simulink model "QRF_fp"  (R2019a)
settings: Solver=VariableStepAuto  StartTime=0.0  StopTime=simulation_stop_time  RelTol=1e-3
values from neighbouring files (symbols this model uses):
  sample_time = 1 / input_sample_freq    (= 1e-06)    [project_main.m]
libraries: simulink x5
settings Model: SimulationMode=accelerator  Creator=ASUAD\sasiddi8  LastModifiedBy=ASUAD\sasiddi8
settings OptimizationCC: BlockReduction=off  ConditionallyExecuteInputs=off  DefaultParameterBehavior=Inlined
settings DebuggingCC: SignalRangeChecking=error  AlgebraicLoopMsg=error  IntegerOverflowMsg=none  ParameterDowncastMsg=none  ParameterOverflowMsg=none  ParameterPrecisionLossMsg=none  IntegerSaturationMsg=none
settings HardwareCC: ProdBitPerPointer=32  ProdBitPerSizeT=32  ProdBitPerPtrDiffT=32  ProdLargestAtomicFloat=None  ProdIntDivRoundTo=Undefined  ProdEndianess=Unspecified  ProdWordSize=32  ProdHWDeviceType=ASIC/FPGA->ASIC/FPGA  TargetBitPerLong=64  TargetBitPerPointer=64  TargetBitPerSizeT=64  TargetBitPerPtrDiffT=64  TargetLongLongMode=on  TargetIntDivRoundTo=Zero  TargetEndianess=LittleEndian  TargetWordSize=64  TargetHWDeviceType=Custom Processor->MATLAB Host Computer  ProdEqTarget=off

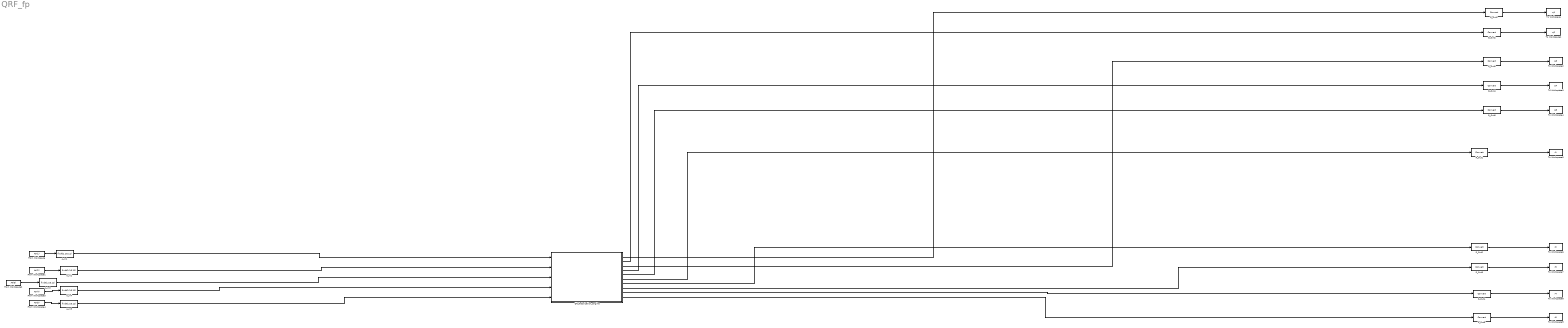
== system QRF_fp ==
  A_In{1..5} (5 alike) : DataTypeConversion  OutDataTypeStr=fixdt(1,16,11)
  From Workspace : FromWorkspace  VariableName=AtI(1)  OutDataTypeStr=double  SampleTime=sample_time  Interpolate=off  OutputAfterFinalValue=Holding final value
  From Workspace1 : FromWorkspace  VariableName=AtI(2)  OutDataTypeStr=double  SampleTime=sample_time  Interpolate=off  OutputAfterFinalValue=Holding final value
  From Workspace2 : FromWorkspace  VariableName=AtI(3)  OutDataTypeStr=double  SampleTime=sample_time  Interpolate=off  OutputAfterFinalValue=Holding final value
  From Workspace3 : FromWorkspace  VariableName=AtI(4)  OutDataTypeStr=double  SampleTime=sample_time  Interpolate=off  OutputAfterFinalValue=Holding final value
  From Workspace4 : FromWorkspace  VariableName=AtI(5)  OutDataTypeStr=double  SampleTime=sample_time  Interpolate=off  OutputAfterFinalValue=Holding final value
  QR_factorization_engine : Subsystem
  Q_Out{1..5} (5 alike) : DataTypeConversion
  R_Out{1..5} (5 alike) : DataTypeConversion
  To Workspace : ToWorkspace  VariableName=q1  SaveFormat=Structure With Time  SampleTime=-1
  To Workspace1 : ToWorkspace  VariableName=q2  SaveFormat=Structure With Time  SampleTime=-1
  To Workspace2 : ToWorkspace  VariableName=q3  SaveFormat=Structure With Time  SampleTime=-1
  To Workspace3 : ToWorkspace  VariableName=q4  SaveFormat=Structure With Time  SampleTime=-1
  To Workspace4 : ToWorkspace  VariableName=q5  SaveFormat=Structure With Time  SampleTime=-1
  To Workspace5 : ToWorkspace  VariableName=r1  SaveFormat=Structure With Time  SampleTime=-1
  To Workspace6 : ToWorkspace  VariableName=r2  SaveFormat=Structure With Time  SampleTime=-1
  To Workspace7 : ToWorkspace  VariableName=r3  SaveFormat=Structure With Time  SampleTime=-1
  To Workspace8 : ToWorkspace  VariableName=r4  SaveFormat=Structure With Time  SampleTime=-1
  To Workspace9 : ToWorkspace  VariableName=r5  SaveFormat=Structure With Time  SampleTime=-1
  wires:
  Q_Out1/1 -> To Workspace/1
  Q_Out2/1 -> To Workspace1/1
  Q_Out3/1 -> To Workspace2/1
  Q_Out4/1 -> To Workspace3/1
  Q_Out5/1 -> To Workspace4/1
  R_Out1/1 -> To Workspace5/1
  R_Out2/1 -> To Workspace6/1
  R_Out3/1 -> To Workspace7/1
  R_Out4/1 -> To Workspace8/1
  R_Out5/1 -> To Workspace9/1
  From Workspace/1 -> A_In1/1
  From Workspace1/1 -> A_In2/1
  From Workspace2/1 -> A_In3/1
  From Workspace3/1 -> A_In4/1
  From Workspace4/1 -> A_In5/1
  A_In1/1 -> QR_factorization_engine/1(In1)
  A_In2/1 -> QR_factorization_engine/2(In2)
  A_In3/1 -> QR_factorization_engine/3(In3)
  A_In4/1 -> QR_factorization_engine/4(In4)
  A_In5/1 -> QR_factorization_engine/5(In5)
  QR_factorization_engine/1(Out1) -> Q_Out1/1
  QR_factorization_engine/2(Out2) -> Q_Out2/1
  QR_factorization_engine/3(Out3) -> Q_Out3/1
  QR_factorization_engine/4(Out4) -> Q_Out4/1
  QR_factorization_engine/5(Out5) -> Q_Out5/1
  QR_factorization_engine/6(Out6) -> R_Out1/1
  QR_factorization_engine/7(Out7) -> R_Out2/1
  QR_factorization_engine/8(Out8) -> R_Out3/1
  QR_factorization_engine/9(Out9) -> R_Out4/1
  QR_factorization_engine/10(Out10) -> R_Out5/1

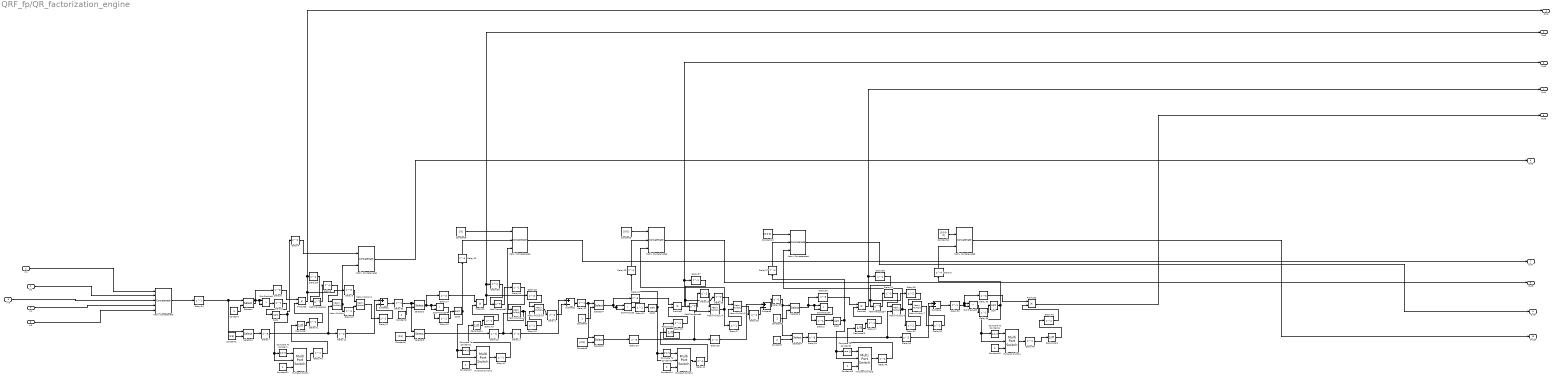
== system QRF_fp/QR_factorization_engine ==
  In1 : Inport
  In2 : Inport  Port=2
  In3 : Inport  Port=3
  In4 : Inport  Port=4
  In5 : Inport  Port=5
  Compare To Constant{,1..4} (5 alike) : simulink/Logic and Bit Operations/Compare To Constant  relop===  const=0  OutDataTypeStr=boolean
  Constant{,2,4,6} (4 alike) : Constant  VectorParams1D=off  OutDataTypeStr=fixdt(0,8,0)  SampleTime=sample_time
  Constant1 : Constant  Value=[2:5]  VectorParams1D=off  OutDataTypeStr=fixdt(0,8,0)  SampleTime=sample_time
  Constant10 : Constant  Value=[0 0 0]  VectorParams1D=off  OutDataTypeStr=fixdt(1,32,26)  SampleTime=sample_time
  Constant11 : Constant  Value=[0 0 0 0]  VectorParams1D=off  OutDataTypeStr=fixdt(0,16,12)  SampleTime=sample_time
  Constant{12..16} (5 alike) : Constant  VectorParams1D=off  OutDataTypeStr=fixdt(0,16,15)  SampleTime=sample_time
  Constant3 : Constant  Value=[2:4]  VectorParams1D=off  OutDataTypeStr=fixdt(0,8,0)  SampleTime=sample_time
  Constant5 : Constant  Value=[2:3]  VectorParams1D=off  OutDataTypeStr=fixdt(0,8,0)  SampleTime=sample_time
  Constant7 : Constant  Value=2  VectorParams1D=off  OutDataTypeStr=fixdt(0,8,0)  SampleTime=sample_time
  Constant8 : Constant  Value=[0]  VectorParams1D=off  OutDataTypeStr=fixdt(1,32,26)  SampleTime=sample_time
  Constant9 : Constant  Value=[0 0]  VectorParams1D=off  OutDataTypeStr=fixdt(1,32,26)  SampleTime=sample_time
  Delay{1..2,5,8,10,12..13,15,19,21,23,27..28,31..33,38,40..58} (36 alike) : Delay  DelayLength=1  InitialCondition=0
  Delay{11,17,25..26,35..36} (6 alike) : Delay  InitialCondition=0
  Delay{6,9,14,18,22,30,39} (7 alike) : Delay  DelayLength=3  InitialCondition=0
  Delay{7,16,24,34} (4 alike) : Delay  DelayLength=5  InitialCondition=0
  Delay{3..4,20,29,37} (5 alike) : Delay  DelayLength=4  InitialCondition=0
  Dot Product{1..4} (4 alike) : DotProduct  OutDataTypeStr=fixdt(0,32,23)
  Dot Product5 : DotProduct  OutDataTypeStr=fixdt(0,32,24)
  MathTranspose{1..4} (4 alike) : Math  Operator=transpose  OutDataTypeStr=double  SaturateOnIntegerOverflow=on
  Matrix Concatenate : Concatenate  NumInputs=5  Mode=Multidimensional array  ConcatenateDimension=2
  Matrix Concatenate1 : Concatenate  Mode=Multidimensional array  ConcatenateDimension=2
  Matrix Concatenate2 : Concatenate  NumInputs=3  Mode=Multidimensional array  ConcatenateDimension=2
  Matrix Concatenate3 : Concatenate  NumInputs=3  Mode=Multidimensional array  ConcatenateDimension=2
  Matrix Concatenate4 : Concatenate  NumInputs=3  Mode=Multidimensional array  ConcatenateDimension=2
  Matrix Concatenate5 : Concatenate  Mode=Multidimensional array  ConcatenateDimension=2
  MatrixMultiply{,2,4,6} (4 alike) : Product  Multiplication=Matrix(*)  OutDataTypeStr=fixdt(1,32,26)
  MatrixMultiply1 : Product  Multiplication=Matrix(*)  OutDataTypeStr=fixdt(1,16,11)
  MatrixMultiply3 : Product  Multiplication=Matrix(*)  OutDataTypeStr=fixdt(1,16,11)
  MatrixMultiply5 : Product  Multiplication=Matrix(*)  OutDataTypeStr=fixdt(1,16,11)
  MatrixMultiply7 : Product  Multiplication=Matrix(*)  OutDataTypeStr=fixdt(1,32,27)
  Multiport Switch{,1..3} (4 alike) : MultiPortSwitch  DataPortOrder=Zero-based contiguous  Inputs=2  zeroidx=on  OutDataTypeStr=fixdt(0,16,11)
  Multiport Switch4 : MultiPortSwitch  DataPortOrder=Zero-based contiguous  Inputs=2  zeroidx=on  OutDataTypeStr=fixdt(0,16,12)
  Product{1..5} (5 alike) : Product  OutDataTypeStr=fixdt(1,16,15)
  Reciprocal : Product  Inputs=/  OutDataTypeStr=fixdt(0,32,31)  SaturateOnIntegerOverflow=on  RndMeth=Zero
  Reciprocal1 : Product  Inputs=/  OutDataTypeStr=fixdt(0,32,31)  SaturateOnIntegerOverflow=on  RndMeth=Zero
  Reciprocal2 : Product  Inputs=/  OutDataTypeStr=fixdt(0,32,30)  SaturateOnIntegerOverflow=on  RndMeth=Zero
  Reciprocal3 : Product  Inputs=/  OutDataTypeStr=fixdt(0,32,29)  SaturateOnIntegerOverflow=on  RndMeth=Zero
  Reciprocal4 : Product  Inputs=/  OutDataTypeStr=fixdt(0,32,25)  SaturateOnIntegerOverflow=on  RndMeth=Zero
  Selector{,1..7} (8 alike) : Selector  NumberOfDimensions=2  InputPortWidth=3  IndexOptions=Select all,Index vector (port)  Indices=[1 3],1  OutputSizes=1,1
  Sqrt : Sqrt  OutDataTypeStr=fixdt(0,16,12)  SaturateOnIntegerOverflow=on
  Sqrt{1..4} (4 alike) : Sqrt  OutDataTypeStr=fixdt(1,32,26)  SaturateOnIntegerOverflow=on
  Subtract1 : Sum  Inputs=+-  AccumDataTypeStr=fixdt(1,32,27)  OutDataTypeStr=fixdt(1,16,11)
  Subtract2 : Sum  Inputs=+-  AccumDataTypeStr=fixdt(1,32,27)  OutDataTypeStr=fixdt(1,16,11)
  Subtract3 : Sum  Inputs=+-  AccumDataTypeStr=fixdt(1,32,27)  OutDataTypeStr=fixdt(1,16,11)
  Subtract4 : Sum  Inputs=+-  AccumDataTypeStr=fixdt(1,32,27)  OutDataTypeStr=fixdt(1,32,27)
  Out1 : Outport
  Out2 : Outport  Port=2
  Out3 : Outport  Port=3
  Out4 : Outport  Port=4
  Out5 : Outport  Port=5
  Out6 : Outport  Port=6
  Out7 : Outport  Port=7
  Out8 : Outport  Port=8
  Out9 : Outport  Port=9
  Out10 : Outport  Port=10
  wires:
  Matrix Concatenate2/1 -> Out7/1
  Compare To Constant/1 -> Multiport Switch/1
  Constant4/1 -> Selector4/2
  Matrix Concatenate3/1 -> Out8/1
  In3/1 -> Matrix Concatenate/3
  MathTranspose2/1 -> Delay15/1
  Compare To Constant2/1 -> Multiport Switch2/1
  Constant8/1 -> Matrix Concatenate2/1
  Selector6/1 -> Dot Product4/2, Dot Product4/1, Delay30/1
  Constant6/1 -> Selector6/2
  Constant16/1 -> Multiport Switch4/3
  MathTranspose3/1 -> Delay23/1
  Matrix Concatenate/1 -> Delay54/1
  Selector7/1 -> Delay34/1
  Constant11/1 -> Matrix Concatenate5/1
  Compare To Constant4/1 -> Multiport Switch4/1
  Selector2/1 -> Dot Product2/2, Dot Product2/1, Delay14/1
  Sqrt1/1 -> Multiport Switch3/2, Compare To Constant3/1, Delay37/1
  Compare To Constant1/1 -> Multiport Switch1/1
  Constant2/1 -> Selector2/2
  In4/1 -> Matrix Concatenate/4
  Sqrt4/1 -> Multiport Switch/2, Compare To Constant/1, Delay4/1
  Sqrt3/1 -> Multiport Switch1/2, Compare To Constant1/1, Delay20/1
  Product4/1 -> Out4/1, Delay58/1
  Product2/1 -> Delay57/1, Out3/1
  MatrixMultiply6/1 -> Delay32/1, Matrix Concatenate4/3
  Constant3/1 -> Selector3/2
  Constant10/1 -> Matrix Concatenate4/1
  Constant12/1 -> Multiport Switch/3
  In1/1 -> Matrix Concatenate/1
  Sqrt/1 -> Multiport Switch4/2, Compare To Constant4/1, Delay3/1
  MatrixMultiply5/1 -> Delay28/1
  Constant1/1 -> Selector1/2
  Selector4/1 -> Dot Product3/1, Dot Product3/2, Delay22/1
  Matrix Concatenate1/1 -> Out6/1
  Selector/1 -> Delay6/1, Dot Product1/2, Dot Product1/1
  In5/1 -> Matrix Concatenate/5
  Dot Product3/1 -> Delay21/1
  Constant7/1 -> Selector7/2
  In2/1 -> Matrix Concatenate/2
  Constant5/1 -> Selector5/2
  Product3/1 -> Delay9/1, Out1/1, Delay55/1
  MatrixMultiply2/1 -> Delay19/1, Matrix Concatenate2/3
  Sqrt2/1 -> Multiport Switch2/2, Compare To Constant2/1, Delay29/1
  Matrix Concatenate5/1 -> Out10/1
  Constant9/1 -> Matrix Concatenate3/1
  Subtract4/1 -> Delay50/1
  Compare To Constant3/1 -> Multiport Switch3/1
  Product5/1 -> Out5/1
  Constant13/1 -> Multiport Switch1/3
  Product1/1 -> Out2/1, Delay56/1, Delay18/1
  Constant/1 -> Selector/2
  Selector5/1 -> Delay24/1
  MatrixMultiply/1 -> Matrix Concatenate1/2, Delay10/1
  Matrix Concatenate4/1 -> Out9/1
  MatrixMultiply4/1 -> Delay27/1, Matrix Concatenate3/3
  Constant15/1 -> Multiport Switch3/3
  Constant14/1 -> Multiport Switch2/3
  Dot Product1/1 -> Delay5/1
  Delay5/1 -> Sqrt4/1
  Delay6/1 -> Product3/1
  MathTranspose1/1 -> Delay8/1
  Delay8/1 -> MatrixMultiply/1
  Selector1/1 -> Delay7/1
  Delay7/1 -> Delay11/1, MatrixMultiply/2
  Delay10/1 -> MatrixMultiply1/2
  Delay9/1 -> MatrixMultiply1/1
  Delay11/1 -> Subtract1/1
  MatrixMultiply1/1 -> Delay12/1
  Delay12/1 -> Subtract1/2
  Delay4/1 -> Matrix Concatenate1/1
  Dot Product2/1 -> Delay13/1
  Delay13/1 -> Sqrt3/1
  Delay14/1 -> Product1/1
  Delay15/1 -> MatrixMultiply2/1
  Selector3/1 -> Delay16/1
  Delay16/1 -> Delay17/1, MatrixMultiply2/2
  Delay17/1 -> Subtract2/1
  Delay18/1 -> MatrixMultiply3/1
  Delay19/1 -> MatrixMultiply3/2
  MatrixMultiply3/1 -> Delay1/1
  Delay1/1 -> Subtract2/2
  Delay20/1 -> Matrix Concatenate2/2
  Delay21/1 -> Sqrt2/1
  Delay22/1 -> Product2/1
  Delay23/1 -> MatrixMultiply4/1
  Delay24/1 -> Delay25/1, MatrixMultiply4/2
  Delay25/1 -> Subtract3/1
  Delay26/1 -> MatrixMultiply5/1
  Delay27/1 -> MatrixMultiply5/2
  Delay28/1 -> Subtract3/2
  Delay29/1 -> Matrix Concatenate3/2
  Delay2/1 -> Sqrt1/1
  Dot Product4/1 -> Delay2/1
  Delay30/1 -> Product4/1
  MathTranspose4/1 -> Delay31/1
  Delay31/1 -> MatrixMultiply6/1
  Delay32/1 -> MatrixMultiply7/2
  MatrixMultiply7/1 -> Delay33/1
  Delay33/1 -> Subtract4/2
  Delay34/1 -> Delay35/1, MatrixMultiply6/2
  Delay35/1 -> Subtract4/1
  Delay36/1 -> MatrixMultiply7/1
  Delay37/1 -> Matrix Concatenate4/2
  Delay38/1 -> Sqrt/1
  Dot Product5/1 -> Delay38/1
  Delay39/1 -> Product5/1
  Delay3/1 -> Matrix Concatenate5/2
  Multiport Switch/1 -> Delay40/1
  Delay40/1 -> Reciprocal/1
  Reciprocal/1 -> Delay41/1
  Delay41/1 -> Product3/2
  Multiport Switch1/1 -> Delay42/1
  Delay42/1 -> Reciprocal1/1
  Reciprocal1/1 -> Delay43/1
  Delay43/1 -> Product1/2
  Multiport Switch2/1 -> Delay44/1
  Delay44/1 -> Reciprocal2/1
  Reciprocal2/1 -> Delay45/1
  Delay45/1 -> Product2/2
  Multiport Switch3/1 -> Delay46/1
  Delay46/1 -> Reciprocal3/1
  Reciprocal3/1 -> Delay47/1
  Delay47/1 -> Product4/2
  Multiport Switch4/1 -> Delay48/1
  Delay48/1 -> Reciprocal4/1
  Reciprocal4/1 -> Delay49/1
  Delay49/1 -> Product5/2
  Delay50/1 -> Dot Product5/2, Delay39/1, Dot Product5/1
  Subtract3/1 -> Delay51/1
  Delay51/1 -> Selector7/1, Selector6/1
  Subtract2/1 -> Delay52/1
  Delay52/1 -> Selector5/1, Selector4/1
  Subtract1/1 -> Delay53/1
  Delay53/1 -> Selector3/1, Selector2/1
  Delay54/1 -> Selector1/1, Selector/1
  Delay55/1 -> MathTranspose1/1
  Delay56/1 -> MathTranspose2/1
  Delay57/1 -> Delay26/1, MathTranspose3/1
  Delay58/1 -> Delay36/1, MathTranspose4/1
